simulink library "AeroLib"  (Simulink 6.0)
settings: Solver=ode45  SolverMode=SingleTasking  StartTime=0.0  StopTime=10.0  RelTol=1e-3
undefined symbols (not defined in the file): Aero, Ap, Atm, Control, Controls, Eng, Flight_cg, Flight_DamperON, Flight_delta_isa, Flight_DeltaSpiral, Flight_InertiaSelect, Flight_ixx, Flight_ixz, Flight_iyy, Flight_izz, Flight_latitude, Flight_LoiterLenght, Flight_LoiterMode, Flight_LoiterRadius, Flight_longitude, Flight_MaxTargetPoints, Flight_SensorsON, Flight_TimeStep, Flight_TowerWind_X, Flight_TowerWind_Y, Flight_TowerWind_Z, Flight_TowerWindON, Flight_Trimming, Flight_TurbON, Flight_weight, Flight_WindGustON, Flight_WindShearON, Flight_ycg, Flight_zcg, Geom, Lgear, Mass, PEG_CDwbnp, PEG_CLht, PEG_CLht_elev, PEG_CLwbnp, PEG_CMht, PEG_CMwbnp, PEG_CNbeta, PEG_CNr, PEG_CNrud, PEG_CRail, PEG_CRbeta, PEG_CRp, PEG_CRrud, PEG_CYbeta, PEG_CYrud, pow, Sensors
libraries: AeroLib x133, simulink3 x49, simulink x37, aerospace x11
(part 4 of 7)

== system AeroLib/Aerodynamics/Aerodynamics_Pioneer/Aero Total ==
  note: The Wind2Stab and Stab2Body blocks were created to deal
      | with the forces seperately, they are different from the
      | WND2STA and STA2BOA blocks contained in the AMS library.
  Cdyn : Inport  Port=1  LatchInput=off
  Alpha_deg : Inport  Port=2  LatchInput=off
  Beta_deg : Inport  Port=3  LatchInput=off
  Qdyn_N : Inport  Port=4  LatchInput=off
  Moments_body : Inport  Port=5  LatchInput=off
  Forces : Inport  Port=6  LatchInput=off
  dcg2ac : Inport  Port=7  LatchInput=off
  Demux1 : Demux  Outputs=3
  Demux4 : Demux  Outputs=3
  Loads : AeroLib/Aerodynamics/Loads  Bref=Geom.Wing.bref  Cref=Geom.Wing.cref  Sw=Geom.Wing.sw
  Selector : Selector  Elements=[1 2 3]  InputPortWidth=6
  Selector1 : Selector  Elements=[4 5 6]  InputPortWidth=6
  Stab2Body : Subsystem
  Sum : Sum  Inputs=|++  SaturateOnIntegerOverflow=on  InputSameDT=on
  Sum1 : Sum  Inputs=|++  SaturateOnIntegerOverflow=on  InputSameDT=on
  Transf to CG : AeroLib/Aerodynamics/Transf to CG  Bref=Geom.Wing.bref  Cref=Geom.Wing.cref
  Wind2Stab : Subsystem
  Xaero : Outport
  Yaero : Outport  Port=2
  Zaero : Outport  Port=3
  Laero : Outport  Port=4
  Maero : Outport  Port=5
  Naero : Outport  Port=6
  CRcg : Outport  Port=7
  CMcg : Outport  Port=8
  CNcg : Outport  Port=9
  wires:
  Cdyn/1 -> Selector/1, Selector1/1
  Transf to CG/6 -> CNcg/1, Loads/7
  Transf to CG/5 -> CMcg/1, Loads/6
  Transf to CG/4 -> CRcg/1, Loads/5
  Transf to CG/3 -> Loads/4
  Transf to CG/2 -> Loads/3
  Transf to CG/1 -> Loads/2
  Moments_body/1 -> Sum1/1
  Demux1/2 -> Transf to CG/2
  Alpha_deg/1 -> Stab2Body/1(Alpha_Deg)
  Qdyn_N/1 -> Loads/1
  Demux1/1 -> Transf to CG/1
  Demux1/3 -> Transf to CG/3
  Loads/1 -> Xaero/1
  Loads/2 -> Yaero/1
  Loads/3 -> Zaero/1
  Loads/4 -> Laero/1
  Loads/5 -> Maero/1
  Loads/6 -> Naero/1
  Selector/1 -> Sum/2
  Wind2Stab/1(Stab_Axis) -> Stab2Body/2(Stab_Axis)
  Selector1/1 -> Sum1/2
  Sum1/1 -> Demux4/1
  Demux4/2 -> Transf to CG/5
  Demux4/1 -> Transf to CG/4
  Demux4/3 -> Transf to CG/6
  Forces/1 -> Wind2Stab/2(Wind_Axis)
  Beta_deg/1 -> Wind2Stab/1(Beta_Deg)
  Sum/1 -> Demux1/1
  Stab2Body/1(Body_Axis) -> Sum/1
  dcg2ac/1 -> Transf to CG/7

== system AeroLib/Aerodynamics/Aerodynamics_Pioneer/Aero_Coefficients ==
  note: Aerodynamics for the Pioneer UAV
      |
      | Wind Tunnel Test Data:
      | Forces with respect to the Wind axis
      | Moments with respect to the Body axis
  From_Control : Inport  Port=1  LatchInput=off
  From_ATM : Inport  Port=2  LatchInput=off
  Bus Selector : BusSelector  DialogController=Simulink.DDGSource_Bus  OutputSignals=Elev_deg,Ail_deg,Rud_deg
  Bus Selector1 : BusSelector  DialogController=Simulink.DDGSource_Bus  OutputSignals=Alpha,Beta
  Drag : Subsystem
  Lift : Subsystem
  Mux : Mux  Inputs=3
  Mux1 : Mux  Inputs=3
  Pitch : Subsystem
  Roll : Subsystem
  SideForce : Subsystem
  Yaw : Subsystem
  Moments_body : Outport
  Forces_wind : Outport  Port=2
  wires:
  Bus Selector1/2 -> SideForce/1(BetaDeg), Yaw/2(BetaDeg), Roll/2(BetaDeg)  "<Beta>"
  Bus Selector1/1 -> Lift/1(AlphaDeg), Yaw/1(AlphaDeg), Pitch/1(AlphaDeg), Drag/1(AlphaDeg), Roll/1(AlphaDeg)  "<Alpha>"
  Bus Selector/3 -> Yaw/4(RudDeg), SideForce/2(RudDeg)  "<Rud_deg>"
  Bus Selector/2 -> Roll/3(AilDeg), Yaw/3(AilDeg), SideForce/3(AilDeg)  "<Ail_deg>"
  Bus Selector/1 -> Drag/2(ElevDeg), Lift/2(ElevDeg), Pitch/2(ElevDeg)  "<Elev_deg>"
  Yaw/1(CN_Total) -> Mux1/3
  Pitch/1(CM_Total) -> Mux1/2
  Roll/1(CR_Total) -> Mux1/1
  Mux1/1 -> Moments_body/1
  From_ATM/1 -> Bus Selector1/1
  Mux/1 -> Forces_wind/1
  From_Control/1 -> Bus Selector/1
  Lift/1(CL_Total) -> Mux/3
  Drag/1(CD_Total) -> Mux/1
  SideForce/1(CY_Total) -> Mux/2

== system AeroLib/Aerodynamics/Aerodynamics_Pioneer/Aero_Dynamic_Coefficients ==
  FromEqm : Inport  Port=1  LatchInput=off
  FromAtm : Inport  Port=2  LatchInput=off
  Aero LatDyn_Coef : Subsystem
  Aero LongDyn_Coef : Subsystem
  Aero NonDim_Rates : AeroLib/Aerodynamics/Aero NonDim_Rates  Bref=Geom.Wing.bref  Cref=Geom.Wing.cref
  Bus Selector : BusSelector  DialogController=Simulink.DDGSource_Bus  OutputSignals=P_rad,Q_rad,R_rad
  Bus Selector1 : BusSelector  DialogController=Simulink.DDGSource_Bus  OutputSignals=AlphaDot,TAS
  Mux : Mux  Inputs=6
  Mux1 : Mux  Inputs=3
  Cdyn : Outport
  wires:
  FromAtm/1 -> Bus Selector1/1
  FromEqm/1 -> Bus Selector/1
  Aero NonDim_Rates/1 -> Aero LatDyn_Coef/1(p_hat)
  Aero NonDim_Rates/2 -> Aero LatDyn_Coef/2(r_hat)
  Mux/1 -> Cdyn/1
  Bus Selector1/1 -> Aero NonDim_Rates/2  "<AlphaDot>"
  Aero LatDyn_Coef/3(CNdyn) -> Mux/6
  Aero LongDyn_Coef/3(CMdyn) -> Mux/5
  Aero LongDyn_Coef/2(CLdyn) -> Mux/3
  Aero LatDyn_Coef/1(CYdyn) -> Mux/2
  Aero LatDyn_Coef/2(CRdyn) -> Mux/4
  Aero LongDyn_Coef/1(CDdyn) -> Mux/1
  Aero NonDim_Rates/3 -> Aero LongDyn_Coef/1(adot_hat)
  Aero NonDim_Rates/4 -> Aero LongDyn_Coef/2(q_hat)
  Bus Selector1/2 -> Aero NonDim_Rates/3  "<TAS>"
  Bus Selector/1 -> Mux1/1  "<P_rad>"
  Bus Selector/2 -> Mux1/2  "<Q_rad>"
  Bus Selector/3 -> Mux1/3  "<R_rad>"
  Mux1/1 -> Aero NonDim_Rates/1

== system AeroLib/Aerodynamics/INIT_Arms/NP ==
  xcg2ac : Inport  Port=1  LatchInput=off
  zcg2ac : Inport  Port=2  LatchInput=off
  Gain : Gain  SaturateOnIntegerOverflow=on
  Mux2 : Mux  Inputs=3
  xvtac2cg : Fcn  Expr=xacnp*Bref-u
  yvtac2cg : Constant  Value=0
  zhtac2cg : Fcn  Expr=zacnp*Bref-u
  dnpac2cg : Outport
  wires:
  Gain/1 -> dnpac2cg/1
  xvtac2cg/1 -> Mux2/1
  yvtac2cg/1 -> Mux2/2
  zhtac2cg/1 -> Mux2/3
  xcg2ac/1 -> xvtac2cg/1
  Mux2/1 -> Gain/1
  zcg2ac/1 -> zhtac2cg/1

== system AeroLib/Aerodynamics/INIT_Arms/htail ==
  xcg2ac : Inport  Port=1  LatchInput=off
  ycg2ac : Inport  Port=2  LatchInput=off
  zcg2ac : Inport  Port=3  LatchInput=off
  Gain : Gain  SaturateOnIntegerOverflow=on
  Mux2 : Mux  Inputs=3
  xhtac2cg : Fcn  Expr=xacht*Cref-u
  yhtac2cg : Fcn  Expr=yacht*Bref-u
  zhtac2cg : Fcn  Expr=zacht*Cref-u
  dhtac2cg : Outport
  wires:
  xhtac2cg/1 -> Mux2/1
  yhtac2cg/1 -> Mux2/2
  zhtac2cg/1 -> Mux2/3
  xcg2ac/1 -> xhtac2cg/1
  ycg2ac/1 -> yhtac2cg/1
  Mux2/1 -> Gain/1
  zcg2ac/1 -> zhtac2cg/1
  Gain/1 -> dhtac2cg/1

== system AeroLib/Aerodynamics/INIT_Arms/vtail ==
  xcg2ac : Inport  Port=1  LatchInput=off
  zcg2ac : Inport  Port=2  LatchInput=off
  Gain : Gain  SaturateOnIntegerOverflow=on
  Mux2 : Mux  Inputs=3
  xvtac2cg : Fcn  Expr=xacvt*Bref-u
  yvtac2cg : Constant  Value=0
  zhtac2cg : Fcn  Expr=zacvt*Bref-u
  dvtac2cg : Outport
  wires:
  zcg2ac/1 -> zhtac2cg/1
  Mux2/1 -> Gain/1
  xcg2ac/1 -> xvtac2cg/1
  zhtac2cg/1 -> Mux2/3
  yvtac2cg/1 -> Mux2/2
  xvtac2cg/1 -> Mux2/1
  Gain/1 -> dvtac2cg/1

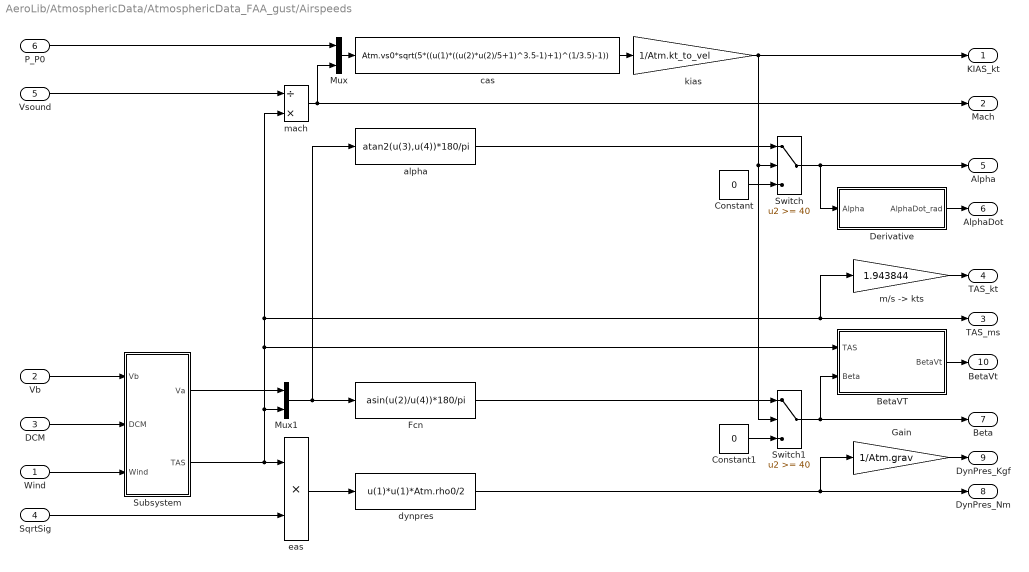
== system AeroLib/AtmosphericData/AtmosphericData_FAA_gust/Airspeeds ==
  Wind : Inport  Port=1  LatchInput=off
  Vb : Inport  Port=2  LatchInput=off
  DCM : Inport  Port=3  LatchInput=off
  SqrtSig : Inport  Port=4  LatchInput=off
  Vsound : Inport  Port=5  LatchInput=off
  P_P0 : Inport  Port=6  LatchInput=off
  BetaVT : Subsystem
  Constant : Constant  Value=0
  Constant1 : Constant  Value=0
  Derivative : Subsystem
  Fcn : Fcn  Expr=asin(u(2)/u(4))*180/pi
  Gain : Gain  Gain=1/Atm.grav  SaturateOnIntegerOverflow=on
  Mux : Mux  Inputs=2
  Mux1 : Mux  Inputs=2
  Subsystem : Subsystem
  Switch : Switch  Threshold=40  SaturateOnIntegerOverflow=on  InputSameDT=on
  Switch1 : Switch  Threshold=40  SaturateOnIntegerOverflow=on  InputSameDT=on
  alpha : Fcn  Expr=atan2(u(3),u(4))*180/pi
  cas : Fcn  Expr=Atm.vs0*sqrt(5*((u(1)*((u(2)*u(2)/5+1)^3.5-1)+1)^(1/3.5)-1))
  dynpres : Fcn  Expr=u(1)*u(1)*Atm.rho0/2
  eas : Product  SaturateOnIntegerOverflow=on  InputSameDT=on
  kias : Gain  Gain=1/Atm.kt_to_vel  SaturateOnIntegerOverflow=on
  "m/s -> kts" : Gain  Gain=1.943844  SaturateOnIntegerOverflow=on
  mach : Product  Inputs=/*  SaturateOnIntegerOverflow=on  InputSameDT=on
  KIAS_kt : Outport
  Mach : Outport  Port=2
  TAS_ms : Outport  Port=3
  TAS_kt : Outport  Port=4
  Alpha : Outport  Port=5
  AlphaDot : Outport  Port=6
  Beta : Outport  Port=7
  DynPres_Nm : Outport  Port=8
  DynPres_Kgf : Outport  Port=9
  BetaVt : Outport  Port=10
  wires:
  Subsystem/1(Va) -> Mux1/1
  "m/s -> kts"/1 -> TAS_kt/1
  Gain/1 -> DynPres_Kgf/1
  Derivative/1(AlphaDot_rad) -> AlphaDot/1
  DCM/1 -> Subsystem/2(DCM)
  Vb/1 -> Subsystem/1(Vb)
  SqrtSig/1 -> eas/2
  eas/1 -> dynpres/1
  Subsystem/2(TAS) -> eas/1, Mux1/2, BetaVT/1(TAS), mach/2, TAS_ms/1, "m/s -> kts"/1
  Vsound/1 -> mach/1
  P_P0/1 -> Mux/1
  mach/1 -> Mux/2, Mach/1
  Mux/1 -> cas/1
  cas/1 -> kias/1
  kias/1 -> KIAS_kt/1, Switch/2, Switch1/2
  alpha/1 -> Switch/1
  Fcn/1 -> Switch1/1
  Constant1/1 -> Switch1/3
  Constant/1 -> Switch/3
  Switch/1 -> Alpha/1, Derivative/1(Alpha)
  Switch1/1 -> Beta/1, BetaVT/2(Beta)
  Wind/1 -> Subsystem/3(Wind)
  BetaVT/1(BetaVt) -> BetaVt/1
  Mux1/1 -> Fcn/1, alpha/1
  dynpres/1 -> DynPres_Nm/1, Gain/1

== system AeroLib/AtmosphericData/AtmosphericData_FAA_gust/Pressure_Altitude ==
  DHpDH : Inport  Port=1  LatchInput=off
  VelI : Inport  Port=2  LatchInput=off
  Fcn1 : Fcn  Expr=-u(1)*u(2)
  FlightTrim_Switch : AeroLib/AMS_StatelessFilters/FlightTrim_Switch
  Gain : Gain  Gain=3.281  SaturateOnIntegerOverflow=on
  Mux : Mux  Inputs=2
  PresAlt : Integrator
  Pres_Alt_ft : Outport  InitialOutput=0
  Hdot_mps : Outport  Port=2
  Pres_Alt_m : Outport  Port=3  InitialOutput=0
  wires:
  FlightTrim_Switch/1 -> Hdot_mps/1, PresAlt/1
  PresAlt/1 -> Pres_Alt_m/1, Gain/1
  DHpDH/1 -> Mux/2
  Mux/1 -> Fcn1/1
  Fcn1/1 -> FlightTrim_Switch/1
  VelI/1 -> Mux/1
  Gain/1 -> Pres_Alt_ft/1

== system AeroLib/AtmosphericData/FAA_Std_Gust/Inputs_to_WindXYZ ==
  note: Horizontal wind direction 0 deg ==> North
      | Horizontal wind direction 90 deg ==> East
      | Horizontal wind direction 180 deg ==> South
      | Horizontal wind direction 270 deg ==> West
      |
      |
      |
      |
      |
      |
      |
      |
      |
      |
      |
      |
      |
      |
      |
      | Vertical wind speed negative ==> Up (ft/s)
      | Vertical wind speed positive ==> Down (ft/s)
  From_Inputs : Inport  Port=1  LatchInput=off
  Bus Selector : BusSelector  DialogController=Simulink.DDGSource_Bus  OutputSignals=Horiz_Wind_Speed,Horiz_Wind_Dir,Vert_Wind_Speed
  Deg-->Rad : Gain  Gain=pi/180  SaturateOnIntegerOverflow=on
  Demux : Demux  Outputs=2
  Mux : Mux  Inputs=2
  Mux1 : Mux  Inputs=3
  Product : Product  SaturateOnIntegerOverflow=on  InputSameDT=on
  Trigonometric Function : Trigonometry  Operator=cos
  Trigonometric Function1 : Trigonometry
  fps-->mps : Gain  Gain=0.3048  SaturateOnIntegerOverflow=on
  kt-->mps : Gain  Gain=0.5144444  SaturateOnIntegerOverflow=on
  Wind_mps : Outport
  wires:
  fps-->mps/1 -> Mux1/3  "WindZ"
  From_Inputs/1 -> Bus Selector/1
  kt-->mps/1 -> Product/1
  Mux1/1 -> Wind_mps/1
  Demux/2 -> Mux1/2  "WindY"
  Demux/1 -> Mux1/1  "WindX"
  Product/1 -> Demux/1
  Bus Selector/1 -> kt-->mps/1  "<Horiz_Wind_Speed>"
  Mux/1 -> Product/2
  Trigonometric Function1/1 -> Mux/2
  Trigonometric Function/1 -> Mux/1
  Deg-->Rad/1 -> Trigonometric Function1/1, Trigonometric Function/1
  Bus Selector/2 -> Deg-->Rad/1  "<Horiz_Wind_Dir>"
  Bus Selector/3 -> fps-->mps/1  "<Vert_Wind_Speed>"

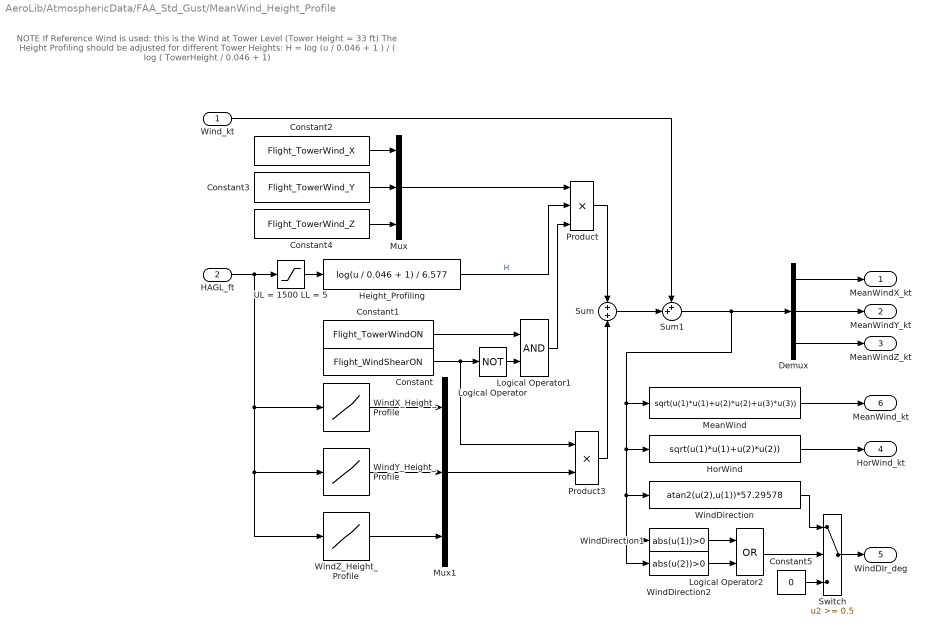
== system AeroLib/AtmosphericData/FAA_Std_Gust/MeanWind_Height_Profile ==
  note: NOTE
      | If Reference Wind is used: this is the Wind at Tower Level (Tower Height = 33 ft)
      | The Height Profiling should be adjusted for different Tower Heights:
      | H = log (u / 0.046 + 1 ) / ( log ( TowerHeight / 0.046 + 1)
  Wind_kt : Inport  Port=1  LatchInput=off
  HAGL_ft : Inport  Port=2  LatchInput=off
  Constant : Constant  Value=Flight_WindShearON
  Constant1 : Constant  Value=Flight_TowerWindON
  Constant2 : Constant  Value=Flight_TowerWind_X
  Constant3 : Constant  Value=Flight_TowerWind_Y
  Constant4 : Constant  Value=Flight_TowerWind_Z
  Constant5 : Constant  Value=0
  Demux : Demux  Outputs=3
  Height_Profiling : Fcn  Expr=log(u / 0.046 + 1) / 6.577
  HorWind : Fcn  Expr=sqrt(u(1)*u(1)+u(2)*u(2))
  Logical Operator : Logic  Operator=NOT
  Logical Operator1 : Logic
  Logical Operator2 : Logic  Operator=OR
  MeanWind : Fcn  Expr=sqrt(u(1)*u(1)+u(2)*u(2)+u(3)*u(3))
  Mux : Mux  Inputs=3
  Mux1 : Mux  Inputs=3
  Product : Product  Inputs=3  SaturateOnIntegerOverflow=on  InputSameDT=on
  Product3 : Product  SaturateOnIntegerOverflow=on  InputSameDT=on
  Sum : Sum  SaturateOnIntegerOverflow=on  InputSameDT=on
  Sum1 : Sum  Inputs=++|  SaturateOnIntegerOverflow=on  InputSameDT=on
  Switch : Switch  Threshold=0.5  SaturateOnIntegerOverflow=on  InputSameDT=on
  UL = 1500 LL = 5 : Saturate  UpperLimit=1500  LowerLimit=5
  WindDirection : Fcn  Expr=atan2(u(2),u(1))*57.29578
  WindDirection1 : Fcn  Expr=abs(u(1))>0
  WindDirection2 : Fcn  Expr=abs(u(2))>0
  WindX_Height_Profile : Lookup  DialogController=Simulink.DDGSource  InputValues=Atm.WindShear.WindHeight  OutputValues=Atm.WindShear.Wind_X  SaturateOnIntegerOverflow=on
  WindY_Height_Profile : Lookup  DialogController=Simulink.DDGSource  InputValues=Atm.WindShear.WindHeight  OutputValues=Atm.WindShear.Wind_Y  SaturateOnIntegerOverflow=on
  WindZ_Height_Profile : Lookup  DialogController=Simulink.DDGSource  InputValues=Atm.WindShear.WindHeight  OutputValues=Atm.WindShear.Wind_Z  SaturateOnIntegerOverflow=on
  MeanWindX_kt : Outport
  MeanWindY_kt : Outport  Port=2
  MeanWindZ_kt : Outport  Port=3
  HorWind_kt : Outport  Port=4
  WindDIr_deg : Outport  Port=5
  MeanWind_kt : Outport  Port=6
  wires:
  Constant5/1 -> Switch/3
  Logical Operator2/1 -> Switch/2
  WindDirection2/1 -> Logical Operator2/2
  WindDirection1/1 -> Logical Operator2/1
  Switch/1 -> WindDIr_deg/1
  WindDirection/1 -> Switch/1
  HorWind/1 -> HorWind_kt/1
  Sum1/1 -> Demux/1, WindDirection2/1, WindDirection1/1, WindDirection/1, HorWind/1, MeanWind/1
  Wind_kt/1 -> Sum1/1
  Demux/3 -> MeanWindZ_kt/1
  Demux/2 -> MeanWindY_kt/1
  Demux/1 -> MeanWindX_kt/1
  MeanWind/1 -> MeanWind_kt/1
  Product3/1 -> Sum/2
  Product/1 -> Sum/1
  Mux1/1 -> Product3/2
  WindZ_Height_Profile/1 -> Mux1/3
  WindY_Height_Profile/1 -> Mux1/2
  WindX_Height_Profile/1 -> Mux1/1
  Logical Operator1/1 -> Product/3
  Height_Profiling/1 -> Product/2  "H"
  Mux/1 -> Product/1
  Constant4/1 -> Mux/3
  Constant3/1 -> Mux/2
  Constant2/1 -> Mux/1
  Constant1/1 -> Logical Operator1/1
  Logical Operator/1 -> Logical Operator1/2
  Constant/1 -> Logical Operator/1, Product3/1
  UL = 1500 LL = 5/1 -> Height_Profiling/1
  HAGL_ft/1 -> WindZ_Height_Profile/1, WindY_Height_Profile/1, WindX_Height_Profile/1, UL = 1500 LL = 5/1
  Sum/1 -> Sum1/2

== system AeroLib/AtmosphericData/FAA_Std_Gust/TASFilter ==
  TAS : Inport  Port=1  LatchInput=off
  Gain : Gain  Gain=50  SaturateOnIntegerOverflow=on
  Sum : Sum  Inputs=|+-  SaturateOnIntegerOverflow=on  InputSameDT=on
  TurbFilter_TAS : Integrator
  TASFilt : Outport
  wires:
  Gain/1 -> TurbFilter_TAS/1
  TurbFilter_TAS/1 -> Sum/2, TASFilt/1
  TAS/1 -> Sum/1
  Sum/1 -> Gain/1  "err"

== system AeroLib/AtmosphericData/FAA_Std_Gust/Turbulence Parameters ==
  Wind_kt : Inport  Port=1  LatchInput=off
  Hagl_ft : Inport  Port=2  LatchInput=off
  TAS_kt : Inport  Port=3  LatchInput=off
  Constant1 : Constant  Value=[0,0,0]
  Constant2 : Constant  Value=Flight_Trimming
  Demux : Demux  Outputs=3
  Hcorr : Fcn  Expr=1/(0.177+.823*u/1000)^0.4
  LH/TAS : Fcn  Expr=600/u
  Mux : Mux  Inputs=3
  Noise_X : RandomNumber  Seed=103956  SampleTime=0
  Noise_Y : RandomNumber  Seed=2938456  SampleTime=0
  Noise_Z : RandomNumber  Seed=33995524  SampleTime=0
  Product : Product  Inputs=*/  SaturateOnIntegerOverflow=on  InputSameDT=on
  Product1 : Product  Inputs=3  SaturateOnIntegerOverflow=on  InputSameDT=on
  Product2 : Product  SaturateOnIntegerOverflow=on  InputSameDT=on
  SC_Factor : Constant  Value=0.0625
  Switch1 : Switch  Threshold=.01  SaturateOnIntegerOverflow=on  InputSameDT=on
  UL = 1000 LL = 1 : Saturate  UpperLimit=1000  LowerLimit=1
  UL = Inf LL = 0.1 : Saturate  UpperLimit=Inf  LowerLimit=0.1
  RMS_h : Outport
  RMS_w : Outport  Port=2
  TLH : Outport  Port=3
  TLW : Outport  Port=4
  Noise_U : Outport  Port=5
  Noise_V : Outport  Port=6
  Noise_W : Outport  Port=7
  wires:
  Demux/3 -> Noise_W/1
  Demux/2 -> Noise_V/1
  Demux/1 -> Noise_U/1
  Constant1/1 -> Switch1/1
  Mux/1 -> Switch1/3
  Constant2/1 -> Switch1/2
  Switch1/1 -> Demux/1
  Noise_Z/1 -> Mux/3
  Noise_Y/1 -> Mux/2
  Noise_X/1 -> Mux/1
  Hagl_ft/1 -> UL = 1000 LL = 1/1
  Wind_kt/1 -> Product2/2, Product1/1
  Product2/1 -> RMS_w/1
  SC_Factor/1 -> Product1/3
  Hcorr/1 -> Product2/1, Product1/2
  Product1/1 -> RMS_h/1
  UL = Inf LL = 0.1/1 -> LH/TAS/1, Product/2  "Tas_kt"
  Product/1 -> TLH/1  "TLH"
  UL = 1000 LL = 1/1 -> Product/1, Hcorr/1  "Hagl"
  LH/TAS/1 -> TLW/1  "TLW"
  TAS_kt/1 -> UL = Inf LL = 0.1/1

== system AeroLib/AtmosphericData/FAA_Std_Gust/Turbulence U ==
  Noise_U : Inport  Port=1  LatchInput=off
  TLH : Inport  Port=2  LatchInput=off
  RMS_h : Inport  Port=3  LatchInput=off
  From_Reset : Inport  Port=4  LatchInput=off
  " (17)" : Product  Inputs=3  SaturateOnIntegerOverflow=on  InputSameDT=on
  (1) : Gain  Gain=6  SaturateOnIntegerOverflow=on
  (12) : Gain  Gain=0.84  SaturateOnIntegerOverflow=on
  (14) : Gain  Gain=0.9186  SaturateOnIntegerOverflow=on
  (15) : Sum  SaturateOnIntegerOverflow=on  InputSameDT=on
  (25) : Gain  Gain=0.0814  SaturateOnIntegerOverflow=on
  Constant : Constant  Value=Flight_TurbON
  Filter Gain (98) Mux_1 : Mux  Inputs=2
  FilterGain : Fcn  Expr=u(1)*sqrt(1/u(2)/pi)
  Filter_U1 : Subsystem
  Filter_U2 : Subsystem
  UL = 30 LL = 0 : Saturate  UpperLimit=30  LowerLimit=0
  UL = 30 LL = 00 : Saturate  UpperLimit=30  LowerLimit=0
  U_turb : Outport
  wires:
  Constant/1 -> " (17)"/3
  TLH/1 -> Filter Gain (98) Mux_1/2, (12)/1, (1)/1  "TLH"
  Noise_U/1 -> Filter_U1/1(Noise), Filter_U2/1(Noise)  "noise_u"
  (14)/1 -> (15)/1
  (25)/1 -> (15)/2
  UL = 30 LL = 00/1 -> Filter_U2/2(Freq)
  UL = 30 LL = 0/1 -> Filter_U1/2(Freq)
  (1)/1 -> UL = 30 LL = 00/1
  (12)/1 -> UL = 30 LL = 0/1
  RMS_h/1 -> Filter Gain (98) Mux_1/1
  (15)/1 -> " (17)"/2  "filter_out"
  FilterGain/1 -> " (17)"/1
  Filter_U2/1(FiltNoise) -> (25)/1  "turb_filter"
  Filter_U1/1(FiltNoise) -> (14)/1  "turb_filter"
  " (17)"/1 -> U_turb/1
  Filter Gain (98) Mux_1/1 -> FilterGain/1
  From_Reset/1 -> Filter_U1/3(From_Reset), Filter_U2/3(From_Reset)

== system AeroLib/AtmosphericData/FAA_Std_Gust/Turbulence V ==
  Noise_V : Inport  Port=1  LatchInput=off
  TLH : Inport  Port=2  LatchInput=off
  RMS_H : Inport  Port=3  LatchInput=off
  From_Reset : Inport  Port=4  LatchInput=off
  " (1)" : Gain  Gain=1.215  SaturateOnIntegerOverflow=on
  " (12)" : Gain  Gain=0.4801  SaturateOnIntegerOverflow=on
  " (14)" : Gain  Gain=0.4161  SaturateOnIntegerOverflow=on
  " (15)" : Sum  Inputs=-++  SaturateOnIntegerOverflow=on  InputSameDT=on
  " (17)" : Product  Inputs=3  SaturateOnIntegerOverflow=on  InputSameDT=on
  " (25)" : Gain  Gain=1.3468  SaturateOnIntegerOverflow=on
  " (44)" : Gain  Gain=0.0693  SaturateOnIntegerOverflow=on
  " (8)" : Gain  Gain=11.14  SaturateOnIntegerOverflow=on
  Constant : Constant  Value=Flight_TurbON
  Filter Gain (98) Mux_1 : Mux  Inputs=2
  FilterGain : Fcn  Expr=u(1)*sqrt(1/u(2)/2/pi)
  Filter_V1 : Subsystem
  Filter_V2 : Subsystem
  Filter_V3 : Subsystem
  Sat1 : Saturate  UpperLimit=30  LowerLimit=0
  Sat2 : Saturate  UpperLimit=30  LowerLimit=0
  Sat3 : Saturate  UpperLimit=30  LowerLimit=0
  V_turb : Outport
  wires:
  Constant/1 -> " (17)"/3
  TLH/1 -> Filter Gain (98) Mux_1/2, " (8)"/1, " (1)"/1, " (12)"/1
  " (14)"/1 -> " (15)"/1
  " (44)"/1 -> " (15)"/3
  Sat3/1 -> Filter_V3/2(Freq)
  Noise_V/1 -> Filter_V2/1(Noise), Filter_V3/1(Noise), Filter_V1/1(Noise)  "noise_v"
  " (15)"/1 -> " (17)"/2
  Sat2/1 -> Filter_V2/2(Freq)
  Sat1/1 -> Filter_V1/2(Freq)
  " (8)"/1 -> Sat3/1
  " (1)"/1 -> Sat2/1
  " (12)"/1 -> Sat1/1
  RMS_H/1 -> Filter Gain (98) Mux_1/1
  Filter_V3/1(FiltNoise) -> " (44)"/1  "turb_filter"
  FilterGain/1 -> " (17)"/1
  " (25)"/1 -> " (15)"/2
  Filter_V2/1(FiltNoise) -> " (25)"/1  "turb_filter"
  Filter_V1/1(FiltNoise) -> " (14)"/1  "turb_filter"
  " (17)"/1 -> V_turb/1
  Filter Gain (98) Mux_1/1 -> FilterGain/1
  From_Reset/1 -> Filter_V1/3(From_Reset), Filter_V2/3(From_Reset), Filter_V3/3(From_Reset)

== system AeroLib/AtmosphericData/FAA_Std_Gust/Turbulence W ==
  Noise_w : Inport  Port=1  LatchInput=off
  TLW : Inport  Port=2  LatchInput=off
  RMS_w : Inport  Port=3  LatchInput=off
  From_Reset : Inport  Port=4  LatchInput=off
  " (1)" : Gain  Gain=1.215  SaturateOnIntegerOverflow=on
  " (12)" : Gain  Gain=0.4801  SaturateOnIntegerOverflow=on
  " (14)" : Gain  Gain=0.4161  SaturateOnIntegerOverflow=on
  " (17)" : Product  Inputs=3  SaturateOnIntegerOverflow=on  InputSameDT=on
  " (25)" : Gain  Gain=1.3468  SaturateOnIntegerOverflow=on
  " (44)" : Gain  Gain=0.0693  SaturateOnIntegerOverflow=on
  " (8)" : Gain  Gain=11.14  SaturateOnIntegerOverflow=on
  (15) : Sum  Inputs=-++  SaturateOnIntegerOverflow=on  InputSameDT=on
  Constant : Constant  Value=Flight_TurbON
  Filter Gain (98) Mux_1 : Mux  Inputs=2
  FilterGain : Fcn  Expr=u(1)*sqrt(1/u(2)/2/pi)
  Filter_W1 : Subsystem
  Filter_W2 : Subsystem
  Filter_W3 : Subsystem
  Sat2 : Saturate  UpperLimit=30  LowerLimit=0
  Sat3 : Saturate  UpperLimit=30  LowerLimit=0
  sat1 : Saturate  UpperLimit=30  LowerLimit=0
  Turb_W : Outport
  wires:
  Constant/1 -> " (17)"/3
  TLW/1 -> Filter Gain (98) Mux_1/2, " (12)"/1, " (8)"/1, " (1)"/1  "TLW"
  Noise_w/1 -> Filter_W2/1(Noise), Filter_W3/1(Noise), Filter_W1/1(Noise)  "noise_w"
  " (14)"/1 -> (15)/1  "Turb_W1"
  Sat3/1 -> Filter_W3/2(Freq)
  Sat2/1 -> Filter_W2/2(Freq)
  sat1/1 -> Filter_W1/2(Freq)
  " (8)"/1 -> Sat3/1
  " (1)"/1 -> Sat2/1
  " (12)"/1 -> sat1/1
  RMS_w/1 -> Filter Gain (98) Mux_1/1  "RMS_w"
  Filter_W3/1(FiltNoise) -> " (44)"/1  "turb_filter"
  (15)/1 -> " (17)"/2
  FilterGain/1 -> " (17)"/1  "t_factor"
  " (44)"/1 -> (15)/3  "Turb_W3"
  " (25)"/1 -> (15)/2  "Turb_W2"
  Filter_W2/1(FiltNoise) -> " (25)"/1  "turb_filter"
  Filter_W1/1(FiltNoise) -> " (14)"/1  "turb_filter"
  " (17)"/1 -> Turb_W/1
  Filter Gain (98) Mux_1/1 -> FilterGain/1
  From_Reset/1 -> Filter_W1/3(From_Reset), Filter_W2/3(From_Reset), Filter_W3/3(From_Reset)

== system AeroLib/Autopilot/Autopilot/AutopilotEngage ==
  From_Inputs : Inport  Port=1  LatchInput=off
  From_Prop : Inport  Port=2  LatchInput=off
  From_FSC : Inport  Port=3  LatchInput=off
  Bus Selector : BusSelector  DialogController=Simulink.DDGSource_Bus  OutputSignals=AutoPilotON,BoosterON
  Bus Selector1 : BusSelector  DialogController=Simulink.DDGSource_Bus  OutputSignals=StopBooster
  Bus Selector2 : BusSelector  DialogController=Simulink.DDGSource_Bus  OutputSignals=FSC_GrSpeed_kt
  Constant4 : Constant  Value=15
  Logical Operator : Logic  Operator=OR
  Logical Operator1 : Logic  Operator=NOT
  Logical Operator2 : Logic  Inputs=3  AllPortsSameDT=off
  Relational Operator : RelationalOperator  Operator=>
  AutopilotON : Outport
  wires:
  Logical Operator2/1 -> AutopilotON/1
  From_FSC/1 -> Bus Selector2/1
  From_Prop/1 -> Bus Selector1/1
  From_Inputs/1 -> Bus Selector/1
  Logical Operator/1 -> Logical Operator2/2
  Relational Operator/1 -> Logical Operator2/3
  Logical Operator1/1 -> Logical Operator/1
  Constant4/1 -> Relational Operator/2
  Bus Selector2/1 -> Relational Operator/1  "<FSC_GrSpeed_kt>"
  Bus Selector/2 -> Logical Operator1/1  "<BoosterON>"
  Bus Selector1/1 -> Logical Operator/2  "<StopBooster>"
  Bus Selector/1 -> Logical Operator2/1  "<AutoPilotON>"

== system AeroLib/Autopilot/Autopilot/Dampers ==
  From_Reset : Inport  Port=1  LatchInput=off
  From_Sen : Inport  Port=2  LatchInput=off
  From_Prop : Inport  Port=3  LatchInput=off
  From_Inputs : Inport  Port=4  LatchInput=off
  Bus Selector : BusSelector  DialogController=Simulink.DDGSource_Bus  OutputSignals=IRU_LatAcc_g
  Bus Selector1 : BusSelector  DialogController=Simulink.DDGSource_Bus  OutputSignals=IRU_Alpha
  Constant1 : Constant  Value=Flight_DamperON
  Constant2 : Constant  Value=[0 0 0]
  Demux : Demux  Outputs=3
  Memory : Memory  X0=[0 0 0]
  Mux : Mux  Inputs=3
  Pitch_Damper : Subsystem
  Roll_Damper : Subsystem
  Switch : Switch  Threshold=0.5  SaturateOnIntegerOverflow=on
  Yaw_Damper : Subsystem
  Elev_cmd : Outport
  Ail_cmd : Outport  Port=2
  Rud_cmd : Outport  Port=3
  wires:
  From_Reset/1 -> Roll_Damper/2(From_Reset), Yaw_Damper/2(From_Reset), Pitch_Damper/1(From_Reset)
  From_Sen/1 -> Pitch_Damper/2(From_INS), Roll_Damper/1(From_Sen), Bus Selector/1, Bus Selector1/1
  From_Prop/1 -> Pitch_Damper/4(From_Prop)
  From_Inputs/1 -> Pitch_Damper/5(From_Inputs)
  Yaw_Damper/1(Rud_cmd) -> Mux/3
  Roll_Damper/1(Ail_cmd) -> Mux/2
  Pitch_Damper/1(Elev_cmd) -> Mux/1
  Bus Selector/1 -> Yaw_Damper/1(Ny)  "<IRU_LatAcc_g>"
  Bus Selector1/1 -> Pitch_Damper/3(Alpha)  "<IRU_Alpha>"
  Constant1/1 -> Switch/2
  Mux/1 -> Memory/1
  Demux/1 -> Elev_cmd/1
  Demux/2 -> Ail_cmd/1
  Demux/3 -> Rud_cmd/1
  Switch/1 -> Demux/1
  Constant2/1 -> Switch/3
  Memory/1 -> Switch/1

== system AeroLib/Autopilot/Autopilot/Guidance ==
  PointsXY : Inport  Port=1  LatchInput=off
  PointsLatLon : Inport  Port=2  LatchInput=off
  From_FSC : Inport  Port=3  LatchInput=off
  From_Prop : Inport  Port=4  LatchInput=off
  From_Reset : Inport  Port=5  LatchInput=off
  From_Inputs : Inport  Port=6  LatchInput=off
  Constant : Constant  Value=Flight_MaxTargetPoints
  Display : Display
  Fcn1 : Fcn  Expr=u(1) < u(2)+0.5
  Loiter_modes : Subsystem
  Look-Up Table : Lookup  DialogController=Simulink.DDGSource  InputValues=[-360 -270 -180-eps -180+eps -90 0 90 180-eps 180+eps 270 360]  OutputValues=[0 90 180 -180 -90 0 90 180 -180 -90 0]  SaturateOnIntegerOverflow=on
  Mux : Mux  Inputs=2
  Switch : Switch  Threshold=0.5  SaturateOnIntegerOverflow=on  InputSameDT=on
  Target_Errors : Subsystem
  Target_Selector : Subsystem
  Terminator : Terminator
  Terminator1 : Terminator
  Speed_Err : Outport
  Track_Err : Outport  Port=2
  Alt_Err : Outport  Port=3
  Bearing : Outport  Port=4
  Time_to_Go : Outport  Port=5
  Point_N : Outport  Port=6
  wires:
  Loiter_modes/2(Point_N) -> Display/1
  Fcn1/1 -> Switch/2
  Loiter_modes/1(Track_Err) -> Switch/3
  Target_Errors/6(Track_Err) -> Switch/1
  Switch/1 -> Look-Up Table/1
  Look-Up Table/1 -> Track_Err/1
  From_FSC/1 -> Target_Errors/7(From_Sen), Loiter_modes/2(From_FSC)
  Target_Errors/1(Distance) -> Target_Selector/1(Distance)
  Target_Selector/4(Z_target) -> Target_Errors/4(Alt_Req)
  Target_Selector/3(V_req) -> Target_Errors/3(Speed_Req)
  Target_Selector/1(Y_target) -> Target_Errors/1(Y_req)
  Target_Selector/2(X_target) -> Target_Errors/2(X_Req)
  Target_Errors/2(Speed_Err) -> Speed_Err/1
  Target_Errors/3(Alt_Err) -> Alt_Err/1
  PointsXY/1 -> Target_Selector/2(PointsXY)
  Target_Errors/4(Bearing) -> Bearing/1
  From_Reset/1 -> Loiter_modes/3(From_Reset), Target_Selector/4(From_Reset)
  From_Prop/1 -> Target_Errors/5(From_Prop)
  From_Inputs/1 -> Target_Errors/6(From_Inputs)
  Mux/1 -> Fcn1/1
  Constant/1 -> Mux/2
  Target_Selector/5(Point_N) -> Loiter_modes/1(Target_N), Mux/1, Point_N/1
  Target_Errors/5(Time_to_Go) -> Time_to_Go/1
  PointsLatLon/1 -> Target_Selector/3(PointsLatLon)
  Target_Selector/6(Lat_target) -> Terminator/1
  Target_Selector/7(Lon_target) -> Terminator1/1

== system AeroLib/Autopilot/Autopilot/PID_AutoPilot ==
  Speed_Err : Inport  Port=1  LatchInput=off
  Track_err : Inport  Port=2  LatchInput=off
  Alt_Err : Inport  Port=3  LatchInput=off
  From_Reset : Inport  Port=4  LatchInput=off
  From_Sen : Inport  Port=5  LatchInput=off
  +-8 : Saturate  UpperLimit=Ap.Track.LimPhi/Ap.Track.err  LowerLimit=-Ap.Track.LimPhi/Ap.Track.err
  Bus Selector : BusSelector  DialogController=Simulink.DDGSource_Bus  OutputSignals=IRU_Phi_deg
  Constant : Constant  Value=0
  Gain : Gain  Gain=Ap.Track.err  SaturateOnIntegerOverflow=on
  PID_Altitude : AeroLib/Autopilot/PID  P=Ap.Alt.pgain  I=Ap.Alt.igain  D=0  Lim_I=Ap.Alt.igainLim  Lim_Err=Ap.Alt.LimAlt  Lim_Com=50
  PID_Throttle : AeroLib/Autopilot/PID  P=Ap.Throttle.pgain  I=Ap.Throttle.igain  D=Ap.Throttle.dgain  Lim_I=Ap.Throttle.igainLim  Lim_Err=50  Lim_Com=1
  PID_Track : AeroLib/Autopilot/PID  P=Ap.Track.pgain  I=0  D=0  Lim_I=1  Lim_Err=50  Lim_Com=Controls.Ail.MaxAngle
  Sum1 : Sum  Inputs=|-+  SaturateOnIntegerOverflow=on  InputSameDT=on
  Elev_cmd : Outport
  Ail_cmd : Outport  Port=2
  Rud_cmd : Outport  Port=3
  Thr_LH_cmd : Outport  Port=4
  Thr_RH_cmd : Outport  Port=5
  wires:
  PID_Altitude/1 -> Elev_cmd/1
  Speed_Err/1 -> PID_Throttle/2
  PID_Throttle/1 -> Thr_LH_cmd/1, Thr_RH_cmd/1
  Constant/1 -> Rud_cmd/1
  PID_Track/1 -> Ail_cmd/1
  Alt_Err/1 -> PID_Altitude/2
  From_Reset/1 -> PID_Altitude/1, PID_Track/1, PID_Throttle/1
  +-8/1 -> Gain/1
  Bus Selector/1 -> Sum1/1  "<IRU_Phi_deg>"
  Gain/1 -> Sum1/2
  From_Sen/1 -> Bus Selector/1
  Track_err/1 -> +-8/1
  Sum1/1 -> PID_Track/2

== system AeroLib/Autopilot/Autopilot/TargetPointsTransform ==
  From_Inputs : Inport  Port=1  LatchInput=off
  Bus Selector : BusSelector  DialogController=Simulink.DDGSource_Bus  OutputSignals=TargetPoints
  GeodCoor to XY : AeroLib/Autopilot/GeodCoor to XY
  Matrix Concatenation : simulink/Math Operations/Matrix Concatenation  numInports=4  catMethod=Horizontal
  Matrix Concatenation1 : simulink/Math Operations/Matrix Concatenation  numInports=2  catMethod=Horizontal
  Reshape{,1..5} (6 alike) : simulink/Math Operations/Reshape  OutputDimensionality=1-D array  OutputDimensions=[1,1]
  Selector : Selector  InputType=Matrix  Elements=[1 3]  Columns=-1  InputPortWidth=3
  Selector1 : Selector  InputType=Matrix  Elements=[1 3]  Rows=2  Columns=-1  InputPortWidth=3
  Selector2 : Selector  InputType=Matrix  Elements=[1 3]  Rows=3  Columns=-1  InputPortWidth=3
  Selector3 : Selector  InputType=Matrix  Elements=[1 3]  Rows=4  Columns=-1  InputPortWidth=3
  TP_XY : Outport
  TP_Lat_Lon : Outport  Port=2
  wires:
  Matrix Concatenation/1 -> TP_XY/1
  GeodCoor to XY/1 -> Reshape/1
  GeodCoor to XY/2 -> Reshape1/1
  GeodCoor to XY/3 -> Reshape2/1
  Selector/1 -> GeodCoor to XY/1, Reshape4/1
  Selector1/1 -> GeodCoor to XY/2, Reshape5/1
  Selector2/1 -> GeodCoor to XY/3
  Selector3/1 -> Reshape3/1
  From_Inputs/1 -> Bus Selector/1
  Bus Selector/1 -> Selector3/1, Selector2/1, Selector/1, Selector1/1  "<TargetPoints>"
  Reshape/1 -> Matrix Concatenation/1
  Reshape1/1 -> Matrix Concatenation/2
  Reshape2/1 -> Matrix Concatenation/3
  Reshape3/1 -> Matrix Concatenation/4
  Matrix Concatenation1/1 -> TP_Lat_Lon/1
  Reshape4/1 -> Matrix Concatenation1/1
  Reshape5/1 -> Matrix Concatenation1/2

== system AeroLib/Autopilot/GeodCoor to XY/Geo2orto ==
  note: Flight_latitude
      | Flight_longitude
      | units are degrees
  Lat_In : Inport  Port=1  LatchInput=off
  Lon_In : Inport  Port=2  LatchInput=off
  Alt_In : Inport  Port=3  LatchInput=off
  Constant : Constant  Value=Flight_latitude
  Constant1 : Constant  Value=6378137
  Constant2 : Constant  Value=Flight_longitude
  Deg-->Rad : Gain  Gain=pi/180  SaturateOnIntegerOverflow=on
  Deg-->Rad1 : Gain  Gain=pi/180  SaturateOnIntegerOverflow=on
  Gain : Gain  Gain=0.5  SaturateOnIntegerOverflow=on
  Gain1 : Gain  Gain=21385  SaturateOnIntegerOverflow=on
  Geod_coor : Subsystem
  Product : Product  SaturateOnIntegerOverflow=on  InputSameDT=on
  Product1 : Product  SaturateOnIntegerOverflow=on  InputSameDT=on
  Sum : Sum  Inputs=|++  SaturateOnIntegerOverflow=on  InputSameDT=on
  Sum1 : Sum  Inputs=|+-  SaturateOnIntegerOverflow=on  InputSameDT=on
  Sum2 : Sum  Inputs=+-+  SaturateOnIntegerOverflow=on  InputSameDT=on
  Trigonometric Function : Trigonometry
  Trigonometric Function7 : Trigonometry  Operator=atan2
  Trigonometric Function8 : Trigonometry  Operator=asin
  X_m : Outport
  Y_m : Outport  Port=2
  wires:
  Deg-->Rad1/1 -> Sum1/2
  Deg-->Rad/1 -> Geod_coor/1(Lat_Init), Sum/1
  Sum2/1 -> Product/1, Product1/1
  Constant/1 -> Deg-->Rad/1
  Sum/1 -> Gain/1
  Gain/1 -> Trigonometric Function/1
  Trigonometric Function/1 -> Gain1/1
  Lat_In/1 -> Sum/2, Geod_coor/2(Lat_Targ)
  Lon_In/1 -> Sum1/1
  Constant2/1 -> Deg-->Rad1/1
  Trigonometric Function8/1 -> Product1/2
  Trigonometric Function7/1 -> Product/2
  Product1/1 -> X_m/1
  Product/1 -> Y_m/1
  Geod_coor/3(Q) -> Trigonometric Function8/1
  Gain1/1 -> Sum2/2
  Constant1/1 -> Sum2/1
  Alt_In/1 -> Sum2/3
  Sum1/1 -> Geod_coor/3(DeltaLon)
  Geod_coor/2(U) -> Trigonometric Function7/2
  Geod_coor/1(P) -> Trigonometric Function7/1

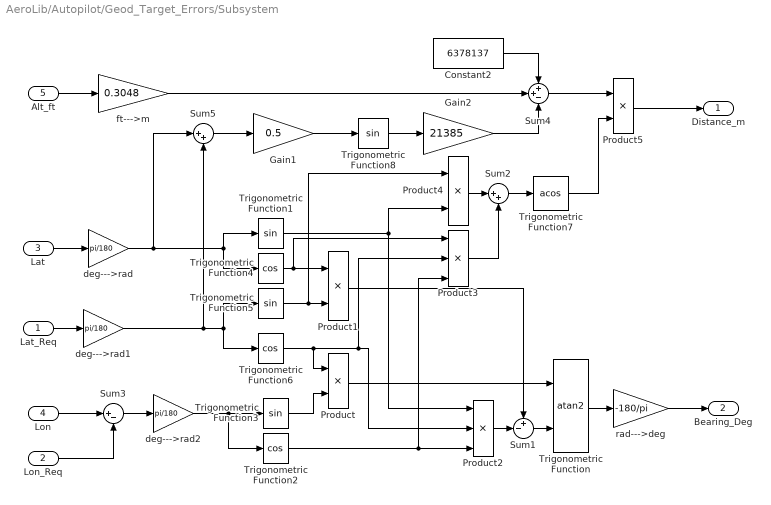
== system AeroLib/Autopilot/Geod_Target_Errors/Subsystem ==
  Lat_Req : Inport  Port=1  LatchInput=off
  Lon_Req : Inport  Port=2  LatchInput=off
  Lat : Inport  Port=3  LatchInput=off
  Lon : Inport  Port=4  LatchInput=off
  Alt_ft : Inport  Port=5  LatchInput=off
  Constant2 : Constant  Value=6378137
  Gain1 : Gain  Gain=0.5  SaturateOnIntegerOverflow=on
  Gain2 : Gain  Gain=21385  SaturateOnIntegerOverflow=on
  Product{,1,4..5} (4 alike) : Product  SaturateOnIntegerOverflow=on  InputSameDT=on
  Product2 : Product  Inputs=3  SaturateOnIntegerOverflow=on  InputSameDT=on
  Product3 : Product  Inputs=3  SaturateOnIntegerOverflow=on  InputSameDT=on
  Sum1 : Sum  Inputs=+-|  SaturateOnIntegerOverflow=on  InputSameDT=on
  Sum2 : Sum  Inputs=|++  SaturateOnIntegerOverflow=on  InputSameDT=on
  Sum3 : Sum  Inputs=|+-  SaturateOnIntegerOverflow=on  InputSameDT=on
  Sum4 : Sum  Inputs=++-  SaturateOnIntegerOverflow=on  InputSameDT=on
  Sum5 : Sum  Inputs=|++  SaturateOnIntegerOverflow=on  InputSameDT=on
  Trigonometric Function : Trigonometry  Operator=atan2
  Trigonometric Function{1,3,5,8} (4 alike) : Trigonometry
  Trigonometric Function2 : Trigonometry  Operator=cos
  Trigonometric Function4 : Trigonometry  Operator=cos
  Trigonometric Function6 : Trigonometry  Operator=cos
  Trigonometric Function7 : Trigonometry  Operator=acos
  deg--->rad : Gain  Gain=pi/180  SaturateOnIntegerOverflow=on
  deg--->rad1 : Gain  Gain=pi/180  SaturateOnIntegerOverflow=on
  deg--->rad2 : Gain  Gain=pi/180  SaturateOnIntegerOverflow=on
  ft--->m : Gain  Gain=0.3048  SaturateOnIntegerOverflow=on
  rad--->deg : Gain  Gain=-180/pi  SaturateOnIntegerOverflow=on
  Distance_m : Outport
  Bearing_Deg : Outport  Port=2
  wires:
  rad--->deg/1 -> Bearing_Deg/1
  Lon/1 -> Sum3/1
  Lon_Req/1 -> Sum3/2
  Sum3/1 -> deg--->rad2/1
  Lat/1 -> deg--->rad/1
  Lat_Req/1 -> deg--->rad1/1
  Trigonometric Function3/1 -> Product/2
  Trigonometric Function6/1 -> Product/1, Product2/2, Product3/2
  Trigonometric Function4/1 -> Product1/1, Product3/1
  Trigonometric Function5/1 -> Product1/2, Product4/1
  Trigonometric Function1/1 -> Product2/1, Product4/2
  Trigonometric Function2/1 -> Product2/3, Product3/3
  Product2/1 -> Sum1/2
  Product1/1 -> Sum1/1
  Product/1 -> Trigonometric Function/1
  Sum1/1 -> Trigonometric Function/2
  Trigonometric Function/1 -> rad--->deg/1
  deg--->rad/1 -> Trigonometric Function1/1, Trigonometric Function4/1, Sum5/1
  deg--->rad1/1 -> Trigonometric Function5/1, Trigonometric Function6/1, Sum5/2
  deg--->rad2/1 -> Trigonometric Function3/1, Trigonometric Function2/1
  Product4/1 -> Sum2/1
  Product3/1 -> Sum2/2
  Sum2/1 -> Trigonometric Function7/1
  Trigonometric Function7/1 -> Product5/2
  Constant2/1 -> Sum4/1
  Trigonometric Function8/1 -> Gain2/1
  Sum4/1 -> Product5/1
  Gain1/1 -> Trigonometric Function8/1
  Sum5/1 -> Gain1/1
  Product5/1 -> Distance_m/1
  Gain2/1 -> Sum4/3
  Alt_ft/1 -> ft--->m/1
  ft--->m/1 -> Sum4/2

== system AeroLib/Controls/Simple_Flap_Actuator/RateLimits ==
  FSLever : Inport  Port=1  LatchInput=off
  Constant : Constant  Value=flap_rate(3)
  Constant1 : Constant  Value=flap_rate(2)
  Constant2 : Constant  Value=flap_rate(1)
  Switch1 : Switch  Threshold=2  SaturateOnIntegerOverflow=on  InputSameDT=on
  Switch21 : Switch  Threshold=5  SaturateOnIntegerOverflow=on  InputSameDT=on
  FlapRate : Outport
  wires:
  FSLever/1 -> Switch21/2, Switch1/2
  Constant/1 -> Switch21/1
  Switch1/1 -> Switch21/3
  Constant1/1 -> Switch1/1
  Constant2/1 -> Switch1/3
  Switch21/1 -> FlapRate/1

== system AeroLib/Controls/Simple_Flap_Actuator/Variable Limiter ==
  Sig : Inport  Port=1  LatchInput=off
  Sat : Inport  Port=2  LatchInput=off
  Gain : Gain  Gain=-1  SaturateOnIntegerOverflow=on
  MinMax : MinMax  Inputs=2  SaturateOnIntegerOverflow=on  InputSameDT=on
  MinMax1 : MinMax  Function=max  Inputs=2  SaturateOnIntegerOverflow=on  InputSameDT=on
  SigSat : Outport
  wires:
  Sig/1 -> MinMax/1
  Sat/1 -> MinMax/2, Gain/1
  MinMax/1 -> MinMax1/1
  Gain/1 -> MinMax1/2
  MinMax1/1 -> SigSat/1

== system AeroLib/Controls/Simple_Flap_Actuator/Variable Limiter1 ==
  Sig : Inport  Port=1  LatchInput=off
  Sat : Inport  Port=2  LatchInput=off
  Gain : Gain  Gain=-1  SaturateOnIntegerOverflow=on
  MinMax : MinMax  Inputs=2  SaturateOnIntegerOverflow=on  InputSameDT=on
  MinMax1 : MinMax  Function=max  Inputs=2  SaturateOnIntegerOverflow=on  InputSameDT=on
  SigSat : Outport
  wires:
  Sig/1 -> MinMax/1
  Sat/1 -> MinMax/2, Gain/1
  MinMax/1 -> MinMax1/1
  Gain/1 -> MinMax1/2
  MinMax1/1 -> SigSat/1

== system AeroLib/CoordinateSystems/QUA2EUL/Bound_2pi ==
  In : Inport  Port=1  LatchInput=off
  2pi : Constant  Value=2*pi
  Math Function : Math  Operator=mod  SaturateOnIntegerOverflow=on
  Out : Outport
  wires:
  Math Function/1 -> Out/1
  2pi/1 -> Math Function/2
  In/1 -> Math Function/1

== system AeroLib/CoordinateSystems/QUA2EUL/Bound_pi ==
  In : Inport  Port=1  LatchInput=off
  2pi : Constant  Value=2*pi
  Math Function : Math  Operator=mod  SaturateOnIntegerOverflow=on
  Sum1 : Sum  Inputs=|+-  SaturateOnIntegerOverflow=on  InputSameDT=on
  Sum2 : Sum  Inputs=|++  SaturateOnIntegerOverflow=on  InputSameDT=on
  pi : Constant  Value=pi
  Out : Outport
  wires:
  Sum1/1 -> Out/1
  pi/1 -> Sum1/2, Sum2/2
  Sum2/1 -> Math Function/1
  In/1 -> Sum2/1
  2pi/1 -> Math Function/2
  Math Function/1 -> Sum1/1

== system AeroLib/CoordinateSystems/QUA2EUL/Bound_pi1 ==
  In : Inport  Port=1  LatchInput=off
  2pi : Constant  Value=2*pi
  Math Function : Math  Operator=mod  SaturateOnIntegerOverflow=on
  Sum1 : Sum  Inputs=|+-  SaturateOnIntegerOverflow=on  InputSameDT=on
  Sum2 : Sum  Inputs=|++  SaturateOnIntegerOverflow=on  InputSameDT=on
  pi : Constant  Value=pi
  Out : Outport
  wires:
  Math Function/1 -> Sum1/1
  2pi/1 -> Math Function/2
  In/1 -> Sum2/1
  Sum2/1 -> Math Function/1
  pi/1 -> Sum2/2, Sum1/2
  Sum1/1 -> Out/1

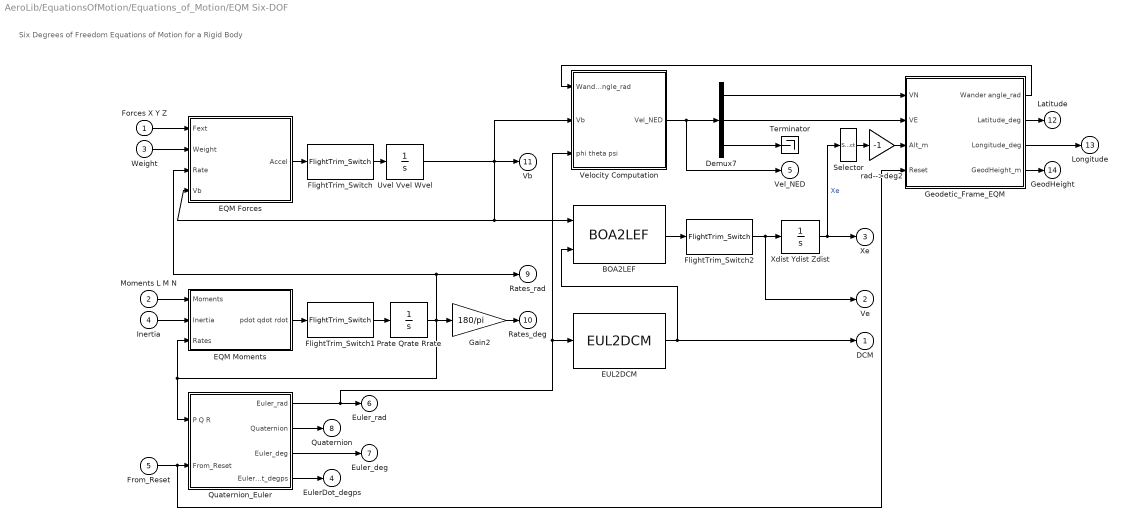
== system AeroLib/EquationsOfMotion/Equations_of_Motion/EQM Six-DOF ==
  note: Six Degrees of Freedom
      | Equations of Motion for a Rigid Body
  Forces X Y Z : Inport  Port=1  LatchInput=off
  Moments L M N : Inport  Port=2  LatchInput=off
  Weight : Inport  Port=3  LatchInput=off
  Inertia : Inport  Port=4  LatchInput=off
  From_Reset : Inport  Port=5  LatchInput=off
  BOA2LEF : AeroLib/CoordinateSystems/BOA2LEF
  Demux7 : Demux  Outputs=3
  EQM Forces : Subsystem
  EQM Moments : Subsystem
  EUL2DCM : AeroLib/CoordinateSystems/EUL2DCM
  FlightTrim_Switch : AeroLib/AMS_StatelessFilters/FlightTrim_Switch
  FlightTrim_Switch1 : AeroLib/AMS_StatelessFilters/FlightTrim_Switch
  FlightTrim_Switch2 : AeroLib/AMS_StatelessFilters/FlightTrim_Switch
  Gain2 : Gain  Gain=180/pi  SaturateOnIntegerOverflow=on
  Geodetic_Frame_EQM : Subsystem
  Prate Qrate Rrate : Integrator
  Quaternion_Euler : Subsystem
  Selector : Selector  Elements=[3]  InputPortWidth=3
  Terminator : Terminator
  Uvel Vvel Wvel : Integrator
  Velocity Computation : Subsystem
  Xdist Ydist Zdist : Integrator
  rad-->deg2 : Gain  Gain=-1  SaturateOnIntegerOverflow=on
  DCM : Outport  InitialOutput=0
  Ve : Outport  Port=2  InitialOutput=0
  Xe : Outport  Port=3  InitialOutput=0
  EulerDot_degps : Outport  Port=4  InitialOutput=0
  Vel_NED : Outport  Port=5  InitialOutput=0
  Euler_rad : Outport  Port=6  InitialOutput=0
  Euler_deg : Outport  Port=7  InitialOutput=0
  Quaternion : Outport  Port=8  InitialOutput=0
  Rates_rad : Outport  Port=9  InitialOutput=0
  Rates_deg : Outport  Port=10  InitialOutput=0
  Vb : Outport  Port=11  InitialOutput=0
  Latitude : Outport  Port=12  InitialOutput=0
  Longitude : Outport  Port=13  InitialOutput=0
  GeodHeight : Outport  Port=14  InitialOutput=0
  wires:
  FlightTrim_Switch1/1 -> Prate Qrate Rrate/1
  FlightTrim_Switch/1 -> Uvel Vvel Wvel/1
  rad-->deg2/1 -> Geodetic_Frame_EQM/3(Alt_m)
  Selector/1 -> rad-->deg2/1
  FlightTrim_Switch2/1 -> Ve/1, Xdist Ydist Zdist/1
  From_Reset/1 -> Geodetic_Frame_EQM/4(Reset), Quaternion_Euler/2(From_Reset)
  Geodetic_Frame_EQM/1(Wander angle_rad) -> Velocity Computation/1(Wander angle_rad)
  Velocity Computation/1(Vel_NED) -> Vel_NED/1, Demux7/1
  Demux7/3 -> Terminator/1
  Quaternion_Euler/4(EulerDot_degps) -> EulerDot_degps/1
  Geodetic_Frame_EQM/2(Latitude_deg) -> Latitude/1
  Geodetic_Frame_EQM/3(Longitude_deg) -> Longitude/1
  Demux7/1 -> Geodetic_Frame_EQM/1(VN)
  Demux7/2 -> Geodetic_Frame_EQM/2(VE)
  Geodetic_Frame_EQM/4(GeodHeight_m) -> GeodHeight/1
  Forces X Y Z/1 -> EQM Forces/1(Fext)
  EQM Moments/1(pdot qdot rdot) -> FlightTrim_Switch1/1
  Moments L M N/1 -> EQM Moments/1(Moments)
  Prate Qrate Rrate/1 -> Gain2/1, EQM Forces/3(Rate), Rates_rad/1, EQM Moments/3(Rates), Quaternion_Euler/1(P Q R)
  Xdist Ydist Zdist/1 -> Selector/1, Xe/1  "Xe"
  EQM Forces/1(Accel) -> FlightTrim_Switch/1
  Uvel Vvel Wvel/1 -> Velocity Computation/2(Vb), EQM Forces/4(Vb), BOA2LEF/1, Vb/1
  Quaternion_Euler/1(Euler_rad) -> Velocity Computation/3(phi theta psi), EUL2DCM/1, Euler_rad/1
  Quaternion_Euler/3(Euler_deg) -> Euler_deg/1
  EUL2DCM/1 -> DCM/1, BOA2LEF/2
  BOA2LEF/1 -> FlightTrim_Switch2/1
  Gain2/1 -> Rates_deg/1
  Inertia/1 -> EQM Moments/2(Inertia)
  Weight/1 -> EQM Forces/2(Weight)
  Quaternion_Euler/2(Quaternion) -> Quaternion/1

== system AeroLib/EquationsOfMotion/Equations_of_Motion/EQM_Outputs ==
  note: m/s_to_kt
  AG_b : Inport  Port=1  LatchInput=off
  DCM : Inport  Port=2  LatchInput=off
  Ve : Inport  Port=3  LatchInput=off
  Xe : Inport  Port=4  LatchInput=off
  AttRates_Degps : Inport  Port=5  LatchInput=off
  Vel_NED : Inport  Port=6  LatchInput=off
  EulerRad : Inport  Port=7  LatchInput=off
  EulerDeg : Inport  Port=8  LatchInput=off
  Quat : Inport  Port=9  LatchInput=off
  RatesRad : Inport  Port=10  LatchInput=off
  RatesDeg : Inport  Port=11  LatchInput=off
  Vb : Inport  Port=12  LatchInput=off
  Latitude : Inport  Port=13  LatchInput=off
  Longitude : Inport  Port=14  LatchInput=off
  GeodHeight : Inport  Port=15  LatchInput=off
  Zext : Inport  Port=16  LatchInput=off
  Mext : Inport  Port=17  LatchInput=off
  NxNyNz : Inport  Port=18  LatchInput=off
  Bus Creator : BusCreator  DialogController=Simulink.DDGSource_Bus  Inputs=48
  Demux{,1..5} (6 alike) : Demux  Outputs=3
  Demux7 : Demux
  Inertilal Positions : Subsystem
  m/s_to_kt1 : Gain  Gain=1.943844  SaturateOnIntegerOverflow=on
  m/s_to_kt2 : Gain  Gain=1.943844  SaturateOnIntegerOverflow=on
  EQM_Out : Outport
  wires:
  DCM/1 -> Inertilal Positions/2(DCM), Bus Creator/2  "DCM"
  AG_b/1 -> Bus Creator/1, Inertilal Positions/1(AG_b)  "AccB"
  Xe/1 -> Inertilal Positions/4(Xe)
  Mext/1 -> Bus Creator/44  "Mext"
  Zext/1 -> Bus Creator/43  "Zext"
  RatesRad/1 -> Demux4/1  "RatesRad"
  Vb/1 -> Bus Creator/45  "Vb"
  Ve/1 -> Bus Creator/3, Inertilal Positions/3(Ve)  "Ve"
  RatesDeg/1 -> Demux1/1
  NxNyNz/1 -> Demux3/1
  EulerDeg/1 -> Demux/1
  Bus Creator/1 -> EQM_Out/1
  EulerRad/1 -> Demux5/1  "EulerRad"
  Demux3/3 -> Bus Creator/42  "Nz"
  Demux3/2 -> Bus Creator/41  "Ny"
  Demux3/1 -> Bus Creator/40  "Nx"
  Demux1/3 -> Bus Creator/39  "R_deg"
  Demux1/2 -> Bus Creator/38  "Q_deg"
  Demux1/1 -> Bus Creator/37  "P_deg"
  Demux/3 -> Bus Creator/29  "Psi_deg"
  Demux/2 -> Bus Creator/28  "The_deg"
  Demux/1 -> Bus Creator/27  "Phi_deg"
  Demux4/3 -> Bus Creator/36  "R_rad"
  Demux4/2 -> Bus Creator/35  "Q_rad"
  Demux4/1 -> Bus Creator/34  "P_rad"
  Demux5/3 -> Bus Creator/26, Inertilal Positions/5(PsiRad)  "Psi_rad"
  Demux5/2 -> Bus Creator/25  "The_rad"
  Demux5/1 -> Bus Creator/24  "Phi_rad"
  Demux7/1 -> Bus Creator/30  "q1"
  Demux7/2 -> Bus Creator/31  "q2"
  Demux7/3 -> Bus Creator/32  "q3"
  Demux7/4 -> Bus Creator/33  "q4"
  Quat/1 -> Demux7/1
  Demux2/3 -> Bus Creator/23  "VD_mps"
  Demux2/2 -> m/s_to_kt2/1
  Demux2/1 -> m/s_to_kt1/1
  m/s_to_kt1/1 -> Bus Creator/21  "VN_kt"
  m/s_to_kt2/1 -> Bus Creator/22  "VE_kt"
  Latitude/1 -> Bus Creator/46  "Latitude"
  Longitude/1 -> Bus Creator/47  "Longitude"
  GeodHeight/1 -> Bus Creator/48  "GeodHeight"
  Inertilal Positions/1(Xdist_m) -> Bus Creator/4  "Xdist_m"
  Inertilal Positions/3(Hagl_m) -> Bus Creator/6  "Hagl_m"
  Inertilal Positions/4(Hagl_ft) -> Bus Creator/7  "Hagl_ft"
  Inertilal Positions/5(Hdot_mps) -> Bus Creator/8  "Hdot_mps"
  Inertilal Positions/7(GroundSpeed_kt) -> Bus Creator/10  "GroundSpeed_kt"
  Inertilal Positions/8(Gamma_deg) -> Bus Creator/11  "Gamma_deg"
  Inertilal Positions/9(Track_deg) -> Bus Creator/12  "Track_deg"
  Inertilal Positions/10(AlongTrackAcc_g) -> Bus Creator/13  "AlongTrackAcc_g"
  Inertilal Positions/11(CrossTrackAcc_g) -> Bus Creator/14  "CrossTrackAcc_g"
  Inertilal Positions/13(AlongPathAcc_g) -> Bus Creator/16  "AlongPathAcc_g"
  Inertilal Positions/14(VertAcc_g) -> Bus Creator/17  "VertAcc_g"
  Inertilal Positions/6(Hdot_ftpmin) -> Bus Creator/9  "Hdot_ftpmin"
  Inertilal Positions/15(AlongHeadAcc_g) -> Bus Creator/18  "AlongHeadAcc_g"
  Inertilal Positions/16(CrossHeadAcc_g) -> Bus Creator/19  "CrossHeadAcc_g"
  Inertilal Positions/12(CrossTrackVel_mps) -> Bus Creator/15  "CrossTrackVel_mps"
  Inertilal Positions/2(Ydist_m) -> Bus Creator/5  "Ydist_m"
  AttRates_Degps/1 -> Bus Creator/20  "AttRates_degps"
  Vel_NED/1 -> Demux2/1

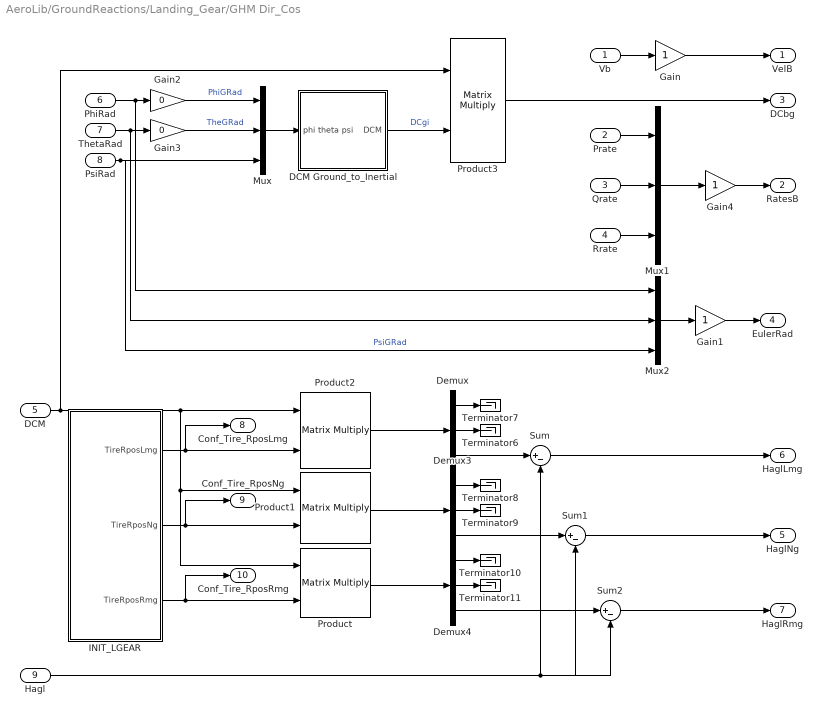
== system AeroLib/GroundReactions/Landing_Gear/GHM Dir_Cos ==
  Vb : Inport  Port=1  LatchInput=off
  Prate : Inport  Port=2  LatchInput=off
  Qrate : Inport  Port=3  LatchInput=off
  Rrate : Inport  Port=4  LatchInput=off
  DCM : Inport  Port=5  LatchInput=off
  PhiRad : Inport  Port=6  LatchInput=off
  ThetaRad : Inport  Port=7  LatchInput=off
  PsiRad : Inport  Port=8  LatchInput=off
  Hagl : Inport  Port=9  LatchInput=off
  DCM Ground_to_Inertial : Subsystem
  Demux : Demux  Outputs=3
  Demux3 : Demux  Outputs=3
  Demux4 : Demux  Outputs=3
  Gain : Gain  SaturateOnIntegerOverflow=on
  Gain1 : Gain  SaturateOnIntegerOverflow=on
  Gain2 : Gain  Gain=0  SaturateOnIntegerOverflow=on
  Gain3 : Gain  Gain=0  SaturateOnIntegerOverflow=on
  Gain4 : Gain  SaturateOnIntegerOverflow=on
  INIT_LGEAR : Subsystem
  Mux : Mux  Inputs=3
  Mux1 : Mux  Inputs=3
  Mux2 : Mux  Inputs=3
  Product{,1..3} (4 alike) : Product  Multiplication=Matrix(*)  SaturateOnIntegerOverflow=on  InputSameDT=on
  Sum : Sum  Inputs=|+-  SaturateOnIntegerOverflow=on  InputSameDT=on
  Sum1 : Sum  Inputs=|+-  SaturateOnIntegerOverflow=on  InputSameDT=on
  Sum2 : Sum  Inputs=|+-  SaturateOnIntegerOverflow=on  InputSameDT=on
  Terminator{6..11} (6 alike) : Terminator
  VelB : Outport
  RatesB : Outport  Port=2
  DCbg : Outport  Port=3
  EulerRad : Outport  Port=4
  HaglNg : Outport  Port=5
  HaglLmg : Outport  Port=6
  HaglRmg : Outport  Port=7
  Conf_Tire_RposLmg : Outport  Port=8
  Conf_Tire_RposNg : Outport  Port=9
  Conf_Tire_RposRmg : Outport  Port=10
  wires:
  Mux/1 -> DCM Ground_to_Inertial/1(phi theta psi)
  Product3/1 -> DCbg/1
  DCM/1 -> Product3/1, Product1/1, Product/1, Product2/1
  Product2/1 -> Demux/1
  DCM Ground_to_Inertial/1(DCM) -> Product3/2  "DCgi"
  Product1/1 -> Demux3/1
  Demux3/1 -> Terminator8/1
  Demux3/2 -> Terminator9/1
  Product/1 -> Demux4/1
  Demux4/1 -> Terminator10/1
  Demux/2 -> Terminator6/1
  Demux4/2 -> Terminator11/1
  Gain/1 -> VelB/1
  Demux/1 -> Terminator7/1
  INIT_LGEAR/1(TireRposLmg) -> Conf_Tire_RposLmg/1, Product2/2
  INIT_LGEAR/2(TireRposNg) -> Conf_Tire_RposNg/1, Product1/2
  INIT_LGEAR/3(TireRposRmg) -> Conf_Tire_RposRmg/1, Product/2
  Vb/1 -> Gain/1
  Prate/1 -> Mux1/1
  Demux/3 -> Sum/1
  Demux3/3 -> Sum1/1
  Sum1/1 -> HaglNg/1
  Sum/1 -> HaglLmg/1
  Demux4/3 -> Sum2/1
  Sum2/1 -> HaglRmg/1
  Hagl/1 -> Sum/2, Sum1/2, Sum2/2
  PhiRad/1 -> Gain2/1, Mux2/1
  Gain2/1 -> Mux/1  "PhiGRad"
  Gain3/1 -> Mux/2  "TheGRad"
  Qrate/1 -> Mux1/2
  Rrate/1 -> Mux1/3
  Mux1/1 -> Gain4/1
  ThetaRad/1 -> Gain3/1, Mux2/2
  PsiRad/1 -> Mux/3, Mux2/3  "PsiGRad"
  Gain4/1 -> RatesB/1
  Mux2/1 -> Gain1/1
  Gain1/1 -> EulerRad/1
